simulink model "VentilatorClosedLoop_gas_f"  (R2018b)
settings: Solver=ode23t  StartTime=0.0  StopTime=50  MaxStep=0.001  RelTol=1e-3  EnableMultiTasking=on
PreLoadFcn:
  | loadVars
values from neighbouring files (symbols this model uses):
  basePSI = 14.7    [loadVars.m]
  D = 0.001    [loadVars.m]
  I = 0.2    [loadVars.m]
  P = 0.2    [loadVars.m]
libraries: fl_lib x26, nesl_utility x9, simulink x2, dspstat3 x1
(part 3 of 3)

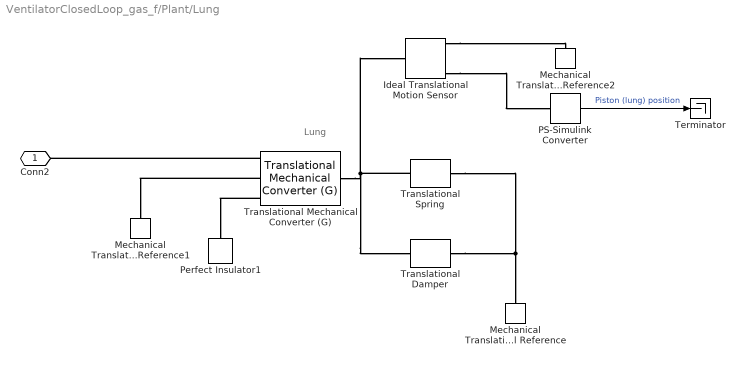
== system VentilatorClosedLoop_gas_f/Plant/Lung ==
  note: Lung
  Ideal Translational Motion Sensor : fl_lib/Mechanical/Mechanical Sensors/Ideal Translational Motion Sensor  offset=0.1 m
  Mechanical Translational Reference : fl_lib/Mechanical/Translational Elements/Mechanical Translational Reference
  Mechanical Translational Reference1 : fl_lib/Mechanical/Translational Elements/Mechanical Translational Reference
  Mechanical Translational Reference2 : fl_lib/Mechanical/Translational Elements/Mechanical Translational Reference
  PS-Simulink Converter : nesl_utility/PS-Simulink Converter  PhysicalDomain=network_engine_domain  SubClassName=ps_output  LeftPortType=input  RightPortType=output  PseudoPeriodic=off  Frequencies=[]  Unit=cm  AffineConversion=off
  Perfect Insulator1 : fl_lib/Thermal/Thermal Elements/Perfect Insulator  T_specify=off  T_priority=None  T=0 K  T_nominal_specify=off  T_nominal_unit=K  T_nominal_value=1
      settings: SourceProductName=Simscape
  Terminator : Terminator
  Translational Mechanical Converter (G) : fl_lib/Gas/Elements/Translational Mechanical Converter (G)  mech_orientation=1  interface_area=4.5 cm^2  length_init=0.1 m  dead_volume=1 cm^3  area_A=0.01 m^2  environment_spec=2  environment_pressure=basePSI psi  p_converter_specify=on  p_converter_priority=High  p_converter=basePSI psi  p_converter_nominal_specify=off  p_converter_nominal_unit=MPa  p_converter_nominal_value=1  T_converter_specify=off  T_converter_priority=High  T_converter=293.15 K  T_converter_nominal_specify=off  T_converter_nominal_unit=K  T_converter_nominal_value=1  rho_converter_specify=off  rho_converter_priority=None  rho_converter=1.2 kg/m^3  rho_converter_nominal_specify=off  rho_converter_nominal_unit=kg/m^3  rho_converter_nominal_value=1
      settings: SourceProductName=Simscape  SourceProductBaseCode=SS
  Translational Damper : fl_lib/Mechanical/Translational Elements/Translational Damper  D=1 lbf/(in/s)  v_specify=off  v_priority=None  v=0 m/s  v_nominal_specify=off  v_nominal_unit=m/s  v_nominal_value=1  f_specify=off  f_priority=None  f=0 N  f_nominal_specify=off  f_nominal_unit=N  f_nominal_value=1
  Translational Spring : fl_lib/Mechanical/Translational Elements/Translational Spring  spr_rate=0.165 lbf/in  v_specify=off  v_priority=None  v=0 m/s  v_nominal_specify=off  v_nominal_unit=m/s  v_nominal_value=1  f_specify=off  f_priority=None  f=0 N  f_nominal_specify=off  f_nominal_unit=N  f_nominal_value=1  x_specify=off  x_priority=High  x=0 m  x_nominal_specify=off  x_nominal_unit=m  x_nominal_value=1
  Conn2 : PMIOPort  Side=Left
  wires:
  PS-Simulink Converter/1 -> Terminator/1  "Piston (lung) position"
  connections:
  Translational Mechanical Converter (G)/LConn2 -- Mechanical Translational Reference1/LConn1
  Ideal Translational Motion Sensor/RConn1 -- Mechanical Translational Reference2/LConn1
  Translational Mechanical Converter (G)/LConn3 -- Perfect Insulator1/LConn1
  Translational Mechanical Converter (G)/LConn1 -- Conn2/RConn1
  Ideal Translational Motion Sensor/RConn3 -- PS-Simulink Converter/LConn1
  Translational Spring/LConn1 -- Translational Mechanical Converter (G)/RConn1 -- Translational Damper/LConn1 -- Ideal Translational Motion Sensor/LConn1
  Translational Spring/RConn1 -- Translational Damper/RConn1 -- Mechanical Translational Reference/LConn1

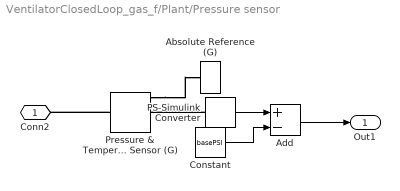
== system VentilatorClosedLoop_gas_f/Plant/Pressure sensor ==
  Absolute Reference (G) : fl_lib/Gas/Elements/Absolute Reference (G)
      settings: SourceProductName=Simscape  SourceProductBaseCode=SS
  Add : Sum  Inputs=+-
  Constant : Constant  Value=basePSI
  PS-Simulink Converter : nesl_utility/PS-Simulink Converter  PhysicalDomain=network_engine_domain  SubClassName=ps_output  LeftPortType=input  RightPortType=output  PseudoPeriodic=off  Frequencies=[]  Unit=psi  AffineConversion=off
  Pressure & Temperature Sensor (G) : fl_lib/Gas/Sensors/Pressure & Temperature Sensor (G)
      settings: SourceProductName=Simscape  SourceProductBaseCode=SS
  Conn2 : PMIOPort  Side=Left
  Out1 : Outport
  wires:
  PS-Simulink Converter/1 -> Add/1
  Constant/1 -> Add/2
  Add/1 -> Out1/1
  connections:
  Pressure & Temperature Sensor (G)/LConn1 -- Conn2/RConn1
  PS-Simulink Converter/LConn1 -- Pressure & Temperature Sensor (G)/RConn2
  Pressure & Temperature Sensor (G)/RConn1 -- Absolute Reference (G)/LConn1

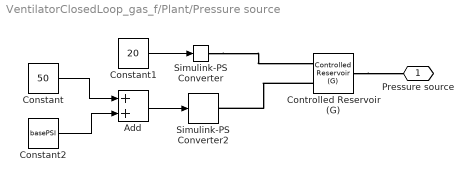
== system VentilatorClosedLoop_gas_f/Plant/Pressure source ==
  Add : Sum
  Constant : Constant  Value=50
  Constant1 : Constant  Value=20
  Constant2 : Constant  Value=basePSI
  Controlled Reservoir (G) : fl_lib/Gas/Elements/Controlled Reservoir (G)  area_A=0.01 m^2
      settings: SourceProductName=Simscape  SourceProductBaseCode=SS
  Simulink-PS Converter : nesl_utility/Simulink-PS Converter  PhysicalDomain=network_engine_domain  SubClassName=ps_input  LeftPortType=input  RightPortType=output  PseudoPeriodic=off  Frequencies=[]  NoiseDistribution=none  NoiseParameters=[]  Unit=degC  AffineConversion=on  FilteringAndDerivatives=provide  SimscapeFilterOrder=1  InputFilterTimeConstant=0.001  UdotUserProvided=0
  Simulink-PS Converter2 : nesl_utility/Simulink-PS Converter  PhysicalDomain=network_engine_domain  SubClassName=ps_input  LeftPortType=input  RightPortType=output  PseudoPeriodic=off  Frequencies=[]  NoiseDistribution=none  NoiseParameters=[]  Unit=psi  AffineConversion=off  FilteringAndDerivatives=zero  SimscapeFilterOrder=1  InputFilterTimeConstant=0.001  UdotUserProvided=1
  Pressure source : PMIOPort  Side=Right
  wires:
  Constant1/1 -> Simulink-PS Converter/1
  Constant2/1 -> Add/2
  Constant/1 -> Add/1
  Add/1 -> Simulink-PS Converter2/1
  connections:
  Controlled Reservoir (G)/LConn1 -- Pressure source/RConn1
  Controlled Reservoir (G)/RConn2 -- Simulink-PS Converter2/RConn1
  Simulink-PS Converter/RConn1 -- Controlled Reservoir (G)/RConn1

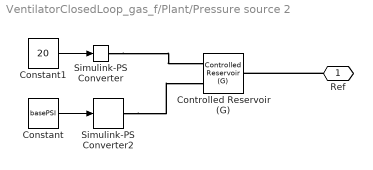
== system VentilatorClosedLoop_gas_f/Plant/Pressure source 2 ==
  Constant : Constant  Value=basePSI
  Constant1 : Constant  Value=20
  Controlled Reservoir (G) : fl_lib/Gas/Elements/Controlled Reservoir (G)  area_A=0.01 m^2
      settings: SourceProductName=Simscape  SourceProductBaseCode=SS
  Simulink-PS Converter : nesl_utility/Simulink-PS Converter  PhysicalDomain=network_engine_domain  SubClassName=ps_input  LeftPortType=input  RightPortType=output  PseudoPeriodic=off  Frequencies=[]  NoiseDistribution=none  NoiseParameters=[]  Unit=degC  AffineConversion=on  FilteringAndDerivatives=provide  SimscapeFilterOrder=1  InputFilterTimeConstant=0.001  UdotUserProvided=0
  Simulink-PS Converter2 : nesl_utility/Simulink-PS Converter  PhysicalDomain=network_engine_domain  SubClassName=ps_input  LeftPortType=input  RightPortType=output  PseudoPeriodic=off  Frequencies=[]  NoiseDistribution=none  NoiseParameters=[]  Unit=psi  AffineConversion=off  FilteringAndDerivatives=zero  SimscapeFilterOrder=1  InputFilterTimeConstant=0.001  UdotUserProvided=1
  Ref : PMIOPort  Side=Right
  wires:
  Constant/1 -> Simulink-PS Converter2/1
  Constant1/1 -> Simulink-PS Converter/1
  connections:
  Simulink-PS Converter2/RConn1 -- Controlled Reservoir (G)/RConn2
  Ref/RConn1 -- Controlled Reservoir (G)/LConn1
  Simulink-PS Converter/RConn1 -- Controlled Reservoir (G)/RConn1

== matlab function VentilatorClosedLoop_gas_f/Peak Pressure Controller/Peak Detector ==
  data: Cmd input; u input; y output
function y = fcn(Cmd,u)
%#codegen
%function [PP, out] =  peakDetect(X,Atk,Dcy)
if Cmd>=0
    Atk = 0.99;
    Dcy = 0.00001;
else
    Atk = 0.99;
    Dcy = 0.002;
end

 
persistent peak
if isempty(peak)
    peak = u;
end

if u>peak
    peak = Atk * u + (1-Atk)* peak;
else
    peak = Dcy * u + (1-Dcy)*peak;
end

y = peak;

== stateflow chart VentilatorClosedLoop_gas_f/Dashboard/Chart1 ==
  state Low
    en: output = 0.049;
  state High
    en: output = 0;
  (default) -> Low
  Low -> High : after(period*OnPortion, sec)
  High -> Low : after(period*(1-OnPortion), sec)
  data: output output; period input; OnPortion input size=1
